simulink model "Half_Adder"  (R2024a)
settings: Solver=FixedStepDiscrete  StartTime=0.0  StopTime=10.0  FixedStep=1  RelTol=1e-3
settings Model: DataTypeOverride=Off  Creator=muzer  LastModifiedBy=muzer
settings OptimizationCC: BlockReduction=off  ConditionallyExecuteInputs=off  DefaultParameterBehavior=Inlined  InheritOutputTypeSmallerThanSingle=on
settings DebuggingCC: ArtificialAlgebraicLoopMsg=error  SingleTaskRateTransMsg=error
settings HardwareCC: ProdBitPerPointer=32  ProdBitPerSizeT=32  ProdBitPerPtrDiffT=32  ProdLargestAtomicFloat=None  ProdIntDivRoundTo=Undefined  ProdEndianess=Unspecified  ProdWordSize=32  ProdHWDeviceType=ASIC/FPGA->ASIC/FPGA  TargetBitPerPointer=64  TargetBitPerSizeT=64  TargetBitPerPtrDiffT=64  TargetLongLongMode=on  TargetIntDivRoundTo=Zero  TargetEndianess=LittleEndian  TargetWordSize=64  TargetHWDeviceType=Custom Processor->MATLAB Host Computer  ProdEqTarget=off

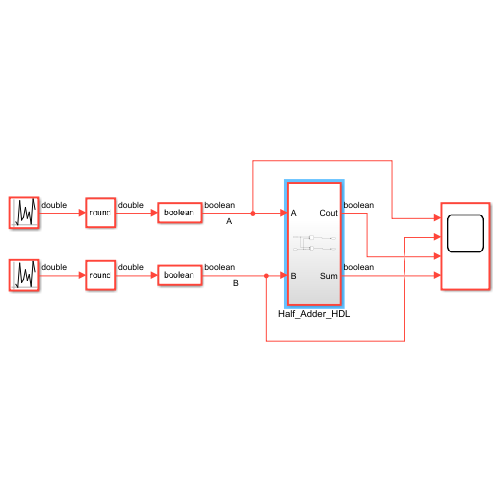
[thumbnail: Simulink's stored preview of the top-level diagram]
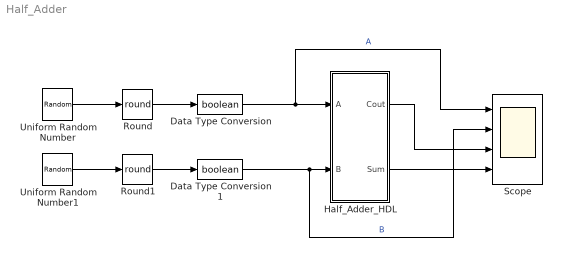
== system Half_Adder ==
  Data Type Conversion : DataTypeConversion  OutDataTypeStr=boolean  SaturateOnIntegerOverflow=off  RndMeth=Floor
  Data Type Conversion1 : DataTypeConversion  OutDataTypeStr=boolean  SaturateOnIntegerOverflow=off  RndMeth=Floor
  Half_Adder_HDL : Subsystem
  Round : Rounding  Operator=round
  Round1 : Rounding  Operator=round
  Scope : Scope  NumInputPorts=4
  Uniform Random Number : UniformRandomNumber  Minimum=0
  Uniform Random Number1 : UniformRandomNumber  Minimum=0  Seed=5
  wires:
  Uniform Random Number/1 -> Round/1
  Round/1 -> Data Type Conversion/1
  Round1/1 -> Data Type Conversion1/1
  Uniform Random Number1/1 -> Round1/1
  Half_Adder_HDL/1(Cout) -> Scope/3
  Half_Adder_HDL/2(Sum) -> Scope/4
  Data Type Conversion/1 -> Scope/1, Half_Adder_HDL/1(A)  "A"
  Data Type Conversion1/1 -> Scope/2, Half_Adder_HDL/2(B)  "B"

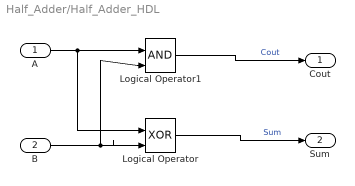
== system Half_Adder/Half_Adder_HDL ==
  A : Inport
  B : Inport  Port=2
  Logical Operator : Logic  Operator=XOR  IconShape=distinctive  AllPortsSameDT=off  OutDataTypeStr=boolean
  Logical Operator1 : Logic  IconShape=distinctive  AllPortsSameDT=off  OutDataTypeStr=boolean
  Cout : Outport
  Sum : Outport  Port=2
  wires:
  B/1 -> Logical Operator/2, Logical Operator1/2
  A/1 -> Logical Operator/1, Logical Operator1/1
  Logical Operator/1 -> Sum/1  "Sum"
  Logical Operator1/1 -> Cout/1  "Cout"
